simulink model "fast_fourier_transform_file"  (R2014b)
settings: Solver=ode23tb  StartTime=0.0  StopTime=0.1  MaxStep=1e-4  RelTol=1e-3
libraries: powerlib x8, powerlib_meascontrol x1
settings Model: Creator=Amr Saleh  LastModifiedBy=Amr Saleh

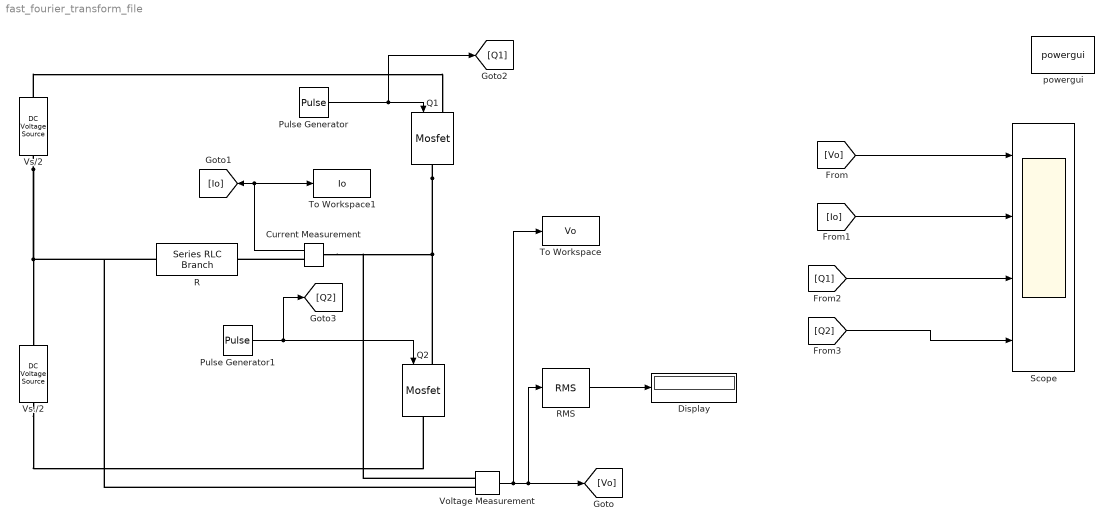
== system fast_fourier_transform_file ==
  Current Measurement : powerlib/Measurements/Current Measurement  PhasorSimulation=off  OutputType=Complex  PSBequivalent=0
  Display : Display
  Pulse Generator : DiscretePulseGenerator  PulseType=Time based  Period=0.02  PulseWidth=50
  Pulse Generator1 : DiscretePulseGenerator  PulseType=Time based  Period=0.02  PulseWidth=50  PhaseDelay=0.01
  Q1 : powerlib/Power Electronics/Mosfet  Ron=0.1  Lon=0  Rd=0.01  Vfd=0  IC=0  Rs=1e5  Cs=inf  Measurements=off
  Q2 : powerlib/Power Electronics/Mosfet  Ron=0.1  Lon=0  Rd=0.01  Vfd=0  IC=0  Rs=1e5  Cs=inf  Measurements=off
  R : powerlib/Elements/Series RLC Branch  LConnTagsString=__new0  RConnTagsString=__new0  BranchType=R  Resistance=5  Inductance=60e-3  SetiL0=off  InitialCurrent=0  Capacitance=1e-6  Setx0=off  InitialVoltage=0  Measurements=None
  RMS : powerlib_meascontrol/Measurements/RMS  TrueRMS=on  Freq=60  RMSInit=120  Ts=0
  Scope : Scope  NumInputPorts=4
      settings: YMin=-30~-5~0~0  YMax=30~5~2~2
  To Workspace : ToWorkspace  VariableName=Vo  SaveFormat=Structure With Time  SampleTime=-1
  To Workspace1 : ToWorkspace  VariableName=Io  SaveFormat=Structure With Time  SampleTime=-1
  Voltage Measurement : powerlib/Measurements/Voltage Measurement  PhasorSimulation=off  OutputType=Complex  PSBequivalent=0
  Vs./2 : powerlib/Electrical Sources/DC Voltage Source  Amplitude=20  Measurements=None
  Vs/2 : powerlib/Electrical Sources/DC Voltage Source  Amplitude=20  Measurements=None
  powergui : powerlib/powergui  Priority=1  SimulationMode=Continuous  SolverType=Tustin/Backward Euler (TBE)  SampleTime=50e-6  frequency=60  SPID=off  DisableSnubberDevices=off  DisableRonSwitches=off  DisableVfSwitches=off  SwTol=0  DisplayEquations=off  Interpol=off  methode=off  Ts=100  frequencyindice=0  Pbase=100e6  ErrMax=1e-4  Iterations=50  UnitsV=kV  UnitsW=MW  FunctionMessages=off  echomessages=off  HookPort=off  EnableUseOfTLC=off  x0status=blocks  RestoreLinks=warning  ResistiveCurrentMeasurement=off  Frange=[0:2:500]  Ylog=off  Xlog=on  ShowGrid=off  save=off  variable=ZData  structure=Io  ZoomFFT=off  StartTime=0.0  cycles=1  DisplayStyle=1  fundamental=50  FreqAxis=on  MaxFrequency=1000  frequencyindicesteady=1  RmsSteady=1  display=off
  wires:
  Voltage Measurement/1 -> To Workspace/1, RMS/1, [Vo]
  Current Measurement/1 -> To Workspace1/1, [Io]
  [Vo] -> Scope/1
  [Io] -> Scope/2
  RMS/1 -> Display/1
  Pulse Generator/1 -> [Q1], Q1/1
  Pulse Generator1/1 -> [Q2], Q2/1
  [Q1] -> Scope/3
  [Q2] -> Scope/4
  connections:
  Vs/2/LConn1 -- Vs./2/RConn1 -- R/LConn1 -- Voltage Measurement/LConn2
  Q1/RConn1 -- Q2/LConn1 -- Current Measurement/LConn1 -- Voltage Measurement/LConn1
  Current Measurement/RConn1 -- R/RConn1
  Vs/2/RConn1 -- Q1/LConn1
  Vs./2/LConn1 -- Q2/RConn1
